simulink model "test_model"  (R2022b)
settings: Solver=VariableStepAuto  StartTime=0.0  StopTime=10.0  RelTol=1e-3
undefined symbols (not defined in the file): DiscIntNeverNeededParam
settings Model: Creator=jorro  LastModifiedBy=JordaoRodolfo
settings ModelReferenceCC: EnableRefExpFcnMdlSchedulingChecks=on

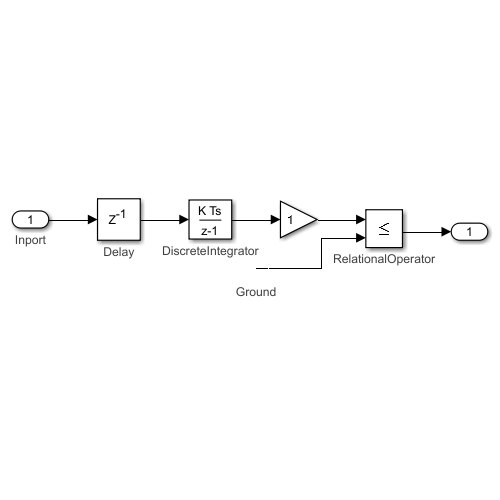
[thumbnail: Simulink's stored preview of the top-level diagram]
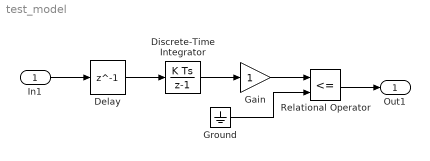
== system test_model ==
  In1 : Inport  SampleTime=2
      settings: AttributesFormatString=%<BlockType>
  Delay : Delay  DelayLength=1  InitialCondition=0
      settings: AttributesFormatString=%<BlockType>
  Discrete-Time Integrator : DiscreteIntegrator  SampleTime=-1  ICPrevOutput=DiscIntNeverNeededParam  ICPrevScaledInput=DiscIntNeverNeededParam
      settings: AttributesFormatString=%<BlockType>
  Gain : Gain
  Ground : Ground
      settings: AttributesFormatString=%<BlockType>
  Relational Operator : RelationalOperator  Operator=<=  OutDataTypeStr=boolean  RndMeth=Simplest  InputSameDT=off
      settings: AttributesFormatString=%<BlockType>
  Out1 : Outport  SampleTime=10
  wires:
  In1/1 -> Delay/1
  Ground/1 -> Relational Operator/2
  Delay/1 -> Discrete-Time Integrator/1
  Discrete-Time Integrator/1 -> Gain/1
  Gain/1 -> Relational Operator/1
  Relational Operator/1 -> Out1/1
